simulink model "Candidacy_Exam_RR"  (R2023a)
settings: Solver=VariableStepAuto  StartTime=0  StopTime=1000  FixedStep=0.01  RelTol=1e-3
model workspace (MAT data in the model file):
  finalint = 0
  firstWarning = 1
  originalScenarioChecksum = '114339432DE22364D47BB28FC96DC10C'
undefined symbols (not defined in the file): Acceleration, ActorID, AngularVelocity, curvature, DefaultGear, Defined, DEND_B, DEND_S, DEND_T, direction, DiscIntNeverNeededParam, driving, Ego, EgoRefPose, gradbp, L, Lane, LF, LR, m, matlabshared, MAX_BRAKE, MAX_STEER, MAX_TORQUE, maxNumActors, MCAR, MIN_BRAKE, MIN_STEER, MIN_TORQUE, n, NUMD_B, NUMD_S, NUMD_T, Pitch, Pose, Position, psi_o, R, Roll, RRdamp, SceneInfo, session, sigbuilder_block, STEER_RATIO, stopSign_ID, Tdead, thetaRefs, TL_ID, TrackWidth, Ts, ts, User, Vdead, Velocity, WB, X_o, xRef2s, Y_o, Yaw, yRef2s
libraries: drivingscenarioandsensors x13, roadrunnerscenario x11, simulink x8, simulink_extras x5, drivingvehiclecontroller x2, trackingutilitieslib x2, robotalgslib x1, mpcadaslib x1, slpidlib x1, drivinglib x1, autolibshared x1, vehdynlibviscommon x1
(part 1 of 5)
settings Model: Creator=akshran  LastModifiedBy=moham
settings DataIOCC: SignalLogging=off
settings OptimizationCC: ReuseModelBlockBuffer=off
settings DebuggingCC: UnconnectedInputMsg=warning  UnconnectedOutputMsg=warning  UnconnectedLineMsg=warning  UnderSpecifiedDimensionMsg=warning
settings ModelReferenceCC: EnableRefExpFcnMdlSchedulingChecks=on
settings RTWCC: DLArmComputeVersion=19.05

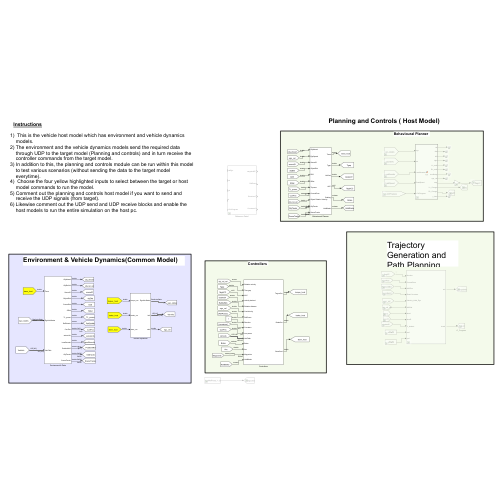
[thumbnail: Simulink's stored preview of the top-level diagram]
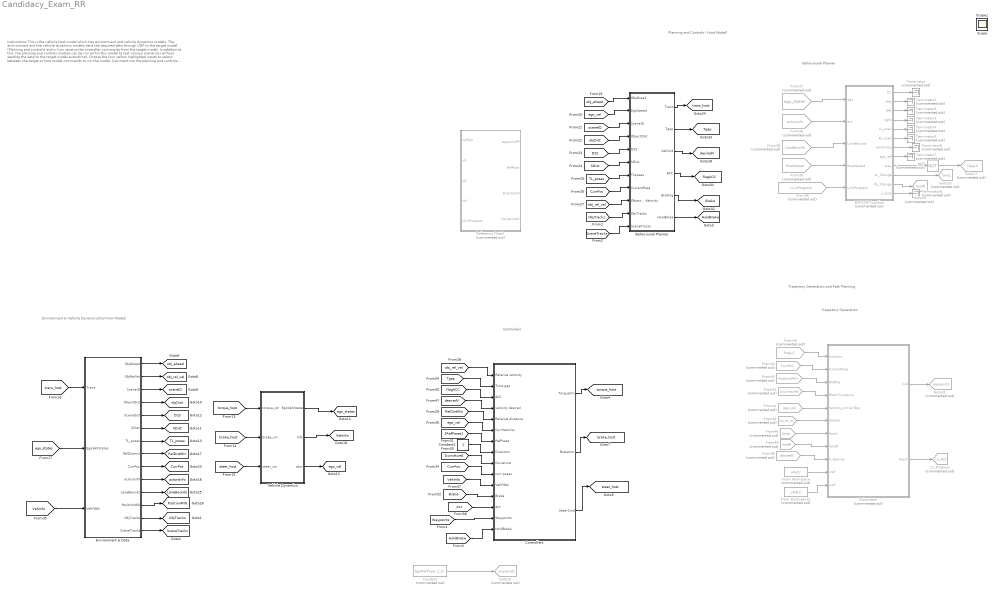
== system Candidacy_Exam_RR ==
  note: Trajectory Generation and Path Planning
  note: Trajectory Generation
  note: Behavioural Planner
  note: Instructions
      |
      | This is the vehicle host model which has environment and vehicle dynamics models.
      | The environment and the vehicle dynamics models send the required data through UDP to the target model (Planning and controls) and in turn receive the controller commands from the target model.
      | In addition to this, the planning and controls module can be run within this model to test various scenarios (without sending the data to the target model everytime).
      | Choose the four yellow highlighted inputs to select between the target or host model commands to run the model.
      | Comment out the planning and controls host model if you want to send and receive the UDP signals (from target).
      | Likewise comment out the UDP send and UDP receive blocks and enable the host models to run the entire simulation on the host pc.
  note: Environment & Vehicle Dynamics(Common Model)
  note: Planning and Controls ( Host Model)
  note: Controllers
  Behavioural Planner : Subsystem
  Constant : Constant  Commented=on  Value=EgoRefPose(:,1:2)
  Constant1 : Constant
  Controllers : Subsystem
  Environment & Data : Subsystem
  From Workspace : FromWorkspace  Commented=on  VariableName=xRef2
  From Workspace1 : FromWorkspace  Commented=on  VariableName=yRef2
  From36 : From  Commented=on  GotoTag=actorsInfo  TagVisibility=global
  From37 : From  Commented=on  GotoTag=ego_states  TagVisibility=global
  From38 : From  Commented=on  GotoTag=LaneBounds  TagVisibility=global
  From39 : From  Commented=on  GotoTag=RoadSpeed  TagVisibility=global
  From40 : From  Commented=on  GotoTag=CurrPos  TagVisibility=global
  From41 : From  Commented=on  GotoTag=curvature
  From42 : From  Commented=on  GotoTag=ego_vel  TagVisibility=global
  From43 : From  Commented=on  GotoTag=PositionMIO  TagVisibility=global
  From44 : From  Commented=on  GotoTag=obj_rel_vel  TagVisibility=global
  From45 : From  Commented=on  GotoTag=flagLC  TagVisibility=global
  From46 : From  Commented=on  GotoTag=laneL  TagVisibility=global
  From48 : From  Commented=on  GotoTag=desiredV  TagVisibility=global
  From49 : From  Commented=on  GotoTag=laneR  TagVisibility=global
  From56 : From  Commented=on  GotoTag=LCinProgress  TagVisibility=global
  Goto19 : Goto  Commented=on  GotoTag=waypoints  TagVisibility=global
  Goto21 : Goto  Commented=on  GotoTag=waypoints  TagVisibility=global
  Goto27 : Goto  Commented=on  GotoTag=flagLC  TagVisibility=global
  Goto29 : Goto  Commented=on  GotoTag=laneL  TagVisibility=global
  Goto30 : Goto  Commented=on  GotoTag=laneR  TagVisibility=global
  LC_Progress : Goto  Commented=on  GotoTag=LC_ACC  TagVisibility=global
  MATLAB Function : MATLAB Function  Commented=on  TreatAsAtomicUnit=on
  NOT : Logic  Commented=on  Operator=NOT  IconShape=distinctive  AllPortsSameDT=off  OutDataTypeStr=boolean
  Reference Data1 : Subsystem  Commented=on  VariantControl=Stanley
  Subsystem : Subsystem  Commented=on
  Terminator{,1..8} (9 alike) : Terminator  Commented=on
  Vehicle Dynamics : Subsystem
  Scope : Scope
  Scope1 : Scope
  tag scope: Brake=global, CurrPos=global, D2S=global, HoldBrake=global, LaneBounds=global, ObjTracks=global, PositionMIO=global, RelDistMin=global, SDist=global, SceneTracks=global, TL_poses=global, Tgap=global, VehInfo=global, actorsInfo=global, brake_host=global, desiredV=global, ego_states=global, ego_vel=global, flagACC=global, objDist=global, obj_ahead=global, obj_rel_vel=global, sceneID=global, steer_host=global, torque_host=global, trans_host=global
  wires:
  Controllers/1(TorgueCm) -> [torque_host]
  Environment & Data/1(ObjAhead) -> [obj_ahead]
  Environment & Data/2(ObjRelVel) -> [obj_rel_vel]
  Environment & Data/3(SceneID) -> [sceneID]
  Environment & Data/4(ObjectDist) -> [objDist]
  Environment & Data/6(SDist) -> [SDist]
  Environment & Data/5(SceneDist) -> [D2S]
  Environment & Data/7(TL_poses) -> [TL_poses]
  Vehicle Dynamics/1(EgoVehStates) -> [ego_states]
  Vehicle Dynamics/3(xdot) -> [ego_vel]
  Environment & Data/8(RelDistmin) -> [RelDistMin]
  Vehicle Dynamics/2(Info) -> [VehInfo]
  [torque_host] -> Vehicle Dynamics/1(torque_cm)
  [brake_host] -> Vehicle Dynamics/2(brake_cm)
  [steer_host] -> Vehicle Dynamics/3(steer_cm)
  [trans_host] -> Environment & Data/1(Trans)
  [ego_states] -> Environment & Data/2(EgoVehStates)
  [obj_rel_vel] -> Controllers/1(Relative velocity)
  [RelDistMin] -> Controllers/5(Relative distance)
  [ego_vel] -> Controllers/6(CurrVelocity)
  [RefPoses] -> Controllers/7(RefPoses)
  Constant1/1 -> Controllers/8(Direction)
  [curvature] -> Controllers/9(Curvature)
  [CurrPos] -> Controllers/10(curr poses)
  [VehInfo] -> Environment & Data/3(VehFdbk)
  Environment & Data/9(CurrPos) -> [CurrPos]
  Environment & Data/10(actorsinfo) -> [actorsInfo]
  From37/1 -> MATLAB Function/1(ego)
  From36/1 -> MATLAB Function/2(act)
  Environment & Data/11(LaneBounds) -> [LaneBounds]
  From38/1 -> MATLAB Function/3(LaneBounds)
  From39/1 -> MATLAB Function/4(RoadSpeed)
  MATLAB Function/9(stay) -> NOT/1
  MATLAB Function/10(LL_Change) -> Goto29/1
  MATLAB Function/11(RL_Change) -> Goto30/1
  Environment & Data/12(PositionMIO) -> [PositionMIO]
  NOT/1 -> Goto27/1
  [desiredV] -> Controllers/4(velocity desired)
  [Tgap] -> Controllers/2(Time gap)
  [flagACC] -> Controllers/3(ACC)
  From56/1 -> MATLAB Function/5(LCinProgress)
  [VehInfo] -> Controllers/11(VehFdbk)
  Controllers/2(BrakeCm) -> [brake_host]
  Controllers/3(SteerCmd) -> [steer_host]
  From45/1 -> Subsystem/1(function)
  From40/1 -> Subsystem/2(CurrentPose)
  From43/1 -> Subsystem/3(MIOPos)
  From41/1 -> Subsystem/4(Road Curvature)
  From42/1 -> Subsystem/5(Velocity_Initial_Ego)
  From44/1 -> Subsystem/6(MIOVel)
  From48/1 -> Subsystem/9(V_desired)
  Subsystem/2(check) -> LC_Progress/1
  [obj_ahead] -> Behavioural Planner/1(ObjAhead)
  [ego_vel] -> Behavioural Planner/2(EgoSpeed)
  [sceneID] -> Behavioural Planner/3(SceneID)
  [objDist] -> Behavioural Planner/4(ObjectDist)
  [D2S] -> Behavioural Planner/5(D2S)
  [SDist] -> Behavioural Planner/6(SDist)
  [TL_poses] -> Behavioural Planner/7(TLposes)
  [CurrPos] -> Behavioural Planner/8(CurrentPose)
  [obj_rel_vel] -> Behavioural Planner/9(Object Relative Velocity)
  Behavioural Planner/1(Trans) -> [trans_host]
  Behavioural Planner/2(Tgap) -> [Tgap]
  Behavioural Planner/3(VelCmd) -> [desiredV]
  Behavioural Planner/4(ACC) -> [flagACC]
  Behavioural Planner/5(Braking) -> [Brake]
  [Brake] -> Controllers/12(Brake)
  [Acc] -> Controllers/13(Acc)
  Subsystem/1(out) -> Goto21/1
  From46/1 -> Subsystem/7(laneL)
  From49/1 -> Subsystem/8(laneR)
  From Workspace/1 -> Subsystem/10(xref)
  From Workspace1/1 -> Subsystem/11(yref)
  MATLAB Function/1(ttc) -> Terminator/1
  MATLAB Function/2(dist) -> Terminator1/1
  MATLAB Function/3(left) -> Terminator2/1
  MATLAB Function/4(right) -> Terminator3/1
  MATLAB Function/5(LL_avail) -> Terminator4/1
  MATLAB Function/6(RL_avail) -> Terminator5/1
  MATLAB Function/7(tend2stay) -> Terminator6/1
  MATLAB Function/8(ego_vel) -> Terminator7/1
  MATLAB Function/12(y_lane) -> Terminator8/1
  Environment & Data/14(SceneTracks) -> [SceneTracks]
  Environment & Data/13(ObjTracks) -> [ObjTracks]
  [ObjTracks] -> Behavioural Planner/10(ObjTracks)
  [SceneTracks] -> Behavioural Planner/11(SceneTracks)
  Behavioural Planner/6(HoldBrake) -> [HoldBrake]
  [HoldBrake] -> Controllers/15(HoldBrake)
  Constant/1 -> Goto19/1
  [Waypoints] -> Controllers/14(Waypoints)

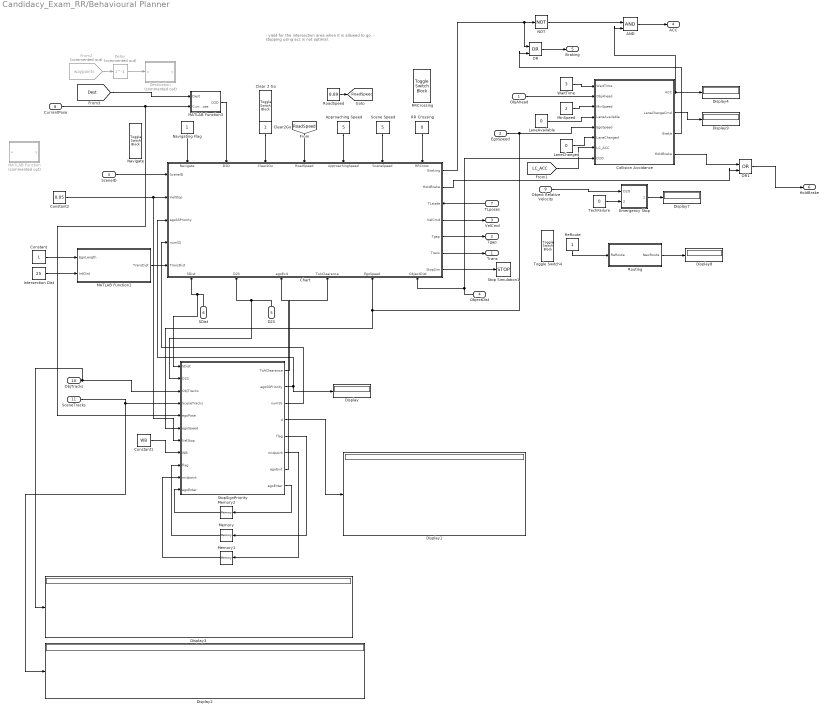
== system Candidacy_Exam_RR/Behavioural Planner ==
  note: - yield for the intersection area when it is allowed to go.
      | - stopping using acc is not optimal.
  ObjAhead : Inport
  EgoSpeed : Inport  Port=2
  SceneID : Inport  Port=3
  ObjectDist : Inport  Port=4
  D2S : Inport  Port=5
  SDist : Inport  Port=6
  TLposes : Inport  Port=7
  CurrentPose : Inport  Port=8
  Object Relative Velocity : Inport  Port=9
  ObjTracks : Inport  Port=10
  SceneTracks : Inport  Port=11
  AND : Logic  IconShape=distinctive  AllPortsSameDT=off  OutDataTypeStr=fixdt(1,16)
  Approaching Speed : Constant  Value=5
  Chart : Stateflow chart  TreatAsAtomicUnit=on
      settings: PortSchema="{\"entries\":[{\"content\":{\"sides\":[{\"content\":{\"connectorIds\":[\"In17\",\"In18\",\"In19\",\"In2\",\"In5\"]},\"type\":\"ConnectorPlacement.EquallySpacedRectSide\",\"uuid\":\"81aca70f-0947-49fb-b60a-be241e44193b\"},{\"content\":{\"connectorIds\":[\"Out6\",\"Out2\",\"In1\",\"Out1\",\"Out3\",\"Out4\",\"Out5\"],\"side\":\"RIGHT\"},\"type\":\"ConnectorPlacement.EquallySpacedRectSide\",\"uuid\":\"e7b9645e-3711-4964-ac9b-0199dd335e99\"},{\"content\":{\"connectorIds\":[\"In13\",\"In14\",\"In15\",\"In16\",\"In6\",\"In9\",\"In11\"],\"side\":\"TOP\"},\"type\":\"ConnectorPlacement.EquallySpacedRectSide\",\"uuid\":\"6876f024-944b-4540-9404-d68f37763657\"},{\"content\":{\"connectorIds\":[\"In10\",\"In12\",\"In3\",\"In4\",\"In7\",\"In8\"],\"side\":\"BOTTOM\"},\"type\":\"ConnectorPlacement.EquallySpacedRectSide\",\"uuid\":\"44acab73-cdde-4edf-95df-27422644ccab\"}]},\"type\":\"ConnectorPlacement.EquallySpacedConnector\",\"uuid\":\"d2c31c01-e447-43db-8d2b-8b98a0ca291a\"}],\"packageUris\":[\"http://schema.mathworks.com/mf0/Connector/R2020b\"],\"version\":\"1.0\"}"
  Clear 2 Go : ToggleSwitchBlock
      settings: Values={{'Off', 'On'}, [0 1]}
  Clear2Go : Constant
  Collision Avoidance : Stateflow chart  TreatAsAtomicUnit=on
  Constant : Constant  Value=L
  Constant1 : Constant  Value=WB
  Constant2 : Constant  Value=0.05
  Delay : Delay  Commented=on  DelayLength=1
  Destination : MATLAB Function  Commented=on  TreatAsAtomicUnit=on
  Display{,1..4,7..9} (8 alike) : Display
  Emergency Stop : Stateflow chart  TreatAsAtomicUnit=on
  From2 : From  Commented=on  GotoTag=waypoints  TagVisibility=global
  Intersection Dist : Constant  Value=25
  LaneAvailable : Constant  Value=0
  LaneChanged : Constant  Value=0
  MATLAB Function : MATLAB Function  Commented=on  TreatAsAtomicUnit=on
  MATLAB Function1 : MATLAB Function  TreatAsAtomicUnit=on
  MATLAB Function3 : MATLAB Function  TreatAsAtomicUnit=on
  Memory : Memory
  Memory1 : Memory  InitialCondition=[0 0]
  Memory2 : Memory
  MinSpeed : Constant  Value=2
  NOT : Logic  Operator=NOT  IconShape=distinctive  AllPortsSameDT=off  OutDataTypeStr=boolean
  Navigate : ToggleSwitchBlock
      settings: Values={{'Off', 'On'}, [0 1]}
  Navigating Flag : Constant
  OR : Logic  Operator=OR  IconShape=distinctive  AllPortsSameDT=off  OutDataTypeStr=boolean
  OR1 : Logic  Operator=OR  IconShape=distinctive  AllPortsSameDT=off  OutDataTypeStr=boolean
  RR Crossing : Constant  Value=0
  RRCrossing : ToggleSwitchBlock
      settings: Values={{'Off', 'On'}, [0 1]}
  ReRoute : Constant
  RoadSpeed : Constant  Value=8.89
  Routing : Stateflow chart  TreatAsAtomicUnit=on
  Scene Speed : Constant  Value=5
  Stop Simulation1 : Stop
  StopSignPriority : MATLAB Function  TreatAsAtomicUnit=on
  TechFailure : Constant  Value=0
  Toggle Switch4 : ToggleSwitchBlock
      settings: Values={{'Off', 'On'}, [0 1]}
  WaitTime : Constant  Value=3
  Trans : Outport
  Tgap : Outport  Port=2
  VelCmd : Outport  Port=3
  ACC : Outport  Port=4
  Braking : Outport  Port=5
  HoldBrake : Outport  Port=6
  tag scope: RoadSpeed=global
  wires:
  Clear2Go/1 -> Chart/15(Clear2Go)
  Routing/1(NewRoute) -> Display8/1
  ObjectDist/1 -> Chart/8(ObjectDist), Collision Avoidance/8(D2O)
  WaitTime/1 -> Collision Avoidance/1(WaitTime)
  Navigating Flag/1 -> Chart/13(Navigate)
  Approaching Speed/1 -> Chart/6(ApproachingSpeed)
  Scene Speed/1 -> Chart/9(SceneSpeed)
  EgoSpeed/1 -> Collision Avoidance/5(EgoSpeed), StopSignPriority/6(egoSpeed), Chart/7(EgoSpeed)
  ReRoute/1 -> Routing/1(ReRoute)
  Collision Avoidance/2(LaneChangeCmd) -> Display9/1
  LaneAvailable/1 -> Collision Avoidance/4(LaneAvailable)
  CurrentPose/1 -> StopSignPriority/5(egoPose), MATLAB Function3/2(CurrentPose)
  RR Crossing/1 -> Chart/11(RRCross)
  MinSpeed/1 -> Collision Avoidance/3(MinSpeed)
  LaneChanged/1 -> Collision Avoidance/6(LaneChanged)
  [RoadSpeed] -> Chart/16(RoadSpeed)
  ObjAhead/1 -> Collision Avoidance/2(ObjAhead)
  SceneID/1 -> Chart/17(SceneID)
  Chart/5(StopSim) -> Stop Simulation1/1
  Chart/4(Trans) -> Trans/1
  TLposes/1 -> Chart/1(TLstate)
  Chart/1(VelCmd) -> VelCmd/1
  SDist/1 -> Chart/10(SDist), StopSignPriority/1(SDist)
  D2S/1 -> Chart/12(D2S), StopSignPriority/2(D2S)
  Chart/3(Tgap) -> Tgap/1
  TechFailure/1 -> Emergency Stop/2(TechFailure)
  Emergency Stop/1(EStop) -> Display7/1
  Object Relative Velocity/1 -> Emergency Stop/1(D2O)
  Collision Avoidance/1(ACC) -> AND/2, Display4/1
  RoadSpeed/1 -> [RoadSpeed]
  NOT/1 -> AND/1
  AND/1 -> ACC/1
  Chart/6(Braking) -> OR/1, NOT/1
  OR/1 -> Braking/1
  Collision Avoidance/3(Brake) -> OR/2
  Constant/1 -> MATLAB Function1/1(EgoLength)
  Intersection Dist/1 -> MATLAB Function1/2(IntDist)
  MATLAB Function1/1(TransDist) -> Chart/5(TransDist)
  [LC_ACC] -> Collision Avoidance/7(LC_ACC)
  From2/1 -> Delay/1
  Delay/1 -> Destination/1(u)
  MATLAB Function3/1(D2D) -> Chart/14(D2D)
  Constant2/1 -> StopSignPriority/7(VelStop), Chart/18(VelStop)
  StopSignPriority/2(egoSSPriority) -> Display/1, Chart/19(egoSSPriority)
  SceneTracks/1 -> Display2/1, StopSignPriority/4(SceneTracks)
  ObjTracks/1 -> Display3/1, StopSignPriority/3(ObjTracks)
  StopSignPriority/3(numSS) -> Chart/2(numSS)
  Constant1/1 -> StopSignPriority/8(WB)
  StopSignPriority/4(d) -> Display1/1
  Memory/1 -> StopSignPriority/9("flag ")
  StopSignPriority/5(flag) -> Memory/1
  StopSignPriority/6(midpoint) -> Memory1/1
  Memory1/1 -> StopSignPriority/10("midpoint ")
  StopSignPriority/7(egoExit) -> Chart/3(egoExit)
  StopSignPriority/1(ToAClearance) -> Chart/4(ToAClearance)
  Chart/2(HoldBrake) -> OR1/2
  StopSignPriority/8(egoEnter) -> Memory2/1
  Memory2/1 -> StopSignPriority/11("egoEnter ")
  OR1/1 -> HoldBrake/1
  Collision Avoidance/4(HoldBrake) -> OR1/1
  [Dest] -> MATLAB Function3/1(Dest)

== system Candidacy_Exam_RR/Controllers ==
  note: Need to write code to get curvature Information
  Relative velocity : Inport
  Time gap : Inport  Port=2
  ACC : Inport  Port=3
  velocity desired : Inport  Port=4
  Relative distance : Inport  Port=5
  CurrVelocity : Inport  Port=6
  RefPoses : Inport  Port=7
  Direction : Inport  Port=8
  Curvature : Inport  Port=9
  curr poses : Inport  Port=10
  VehFdbk : Inport  Port=11
  Brake : Inport  Port=12
  Acc : Inport  Port=13
  Waypoints : Inport  Port=14
  HoldBrake : Inport  Port=15
  Lateral Controllers1 : Subsystem
  Longitudinal Controllers : Subsystem
  MATLAB Function2 : MATLAB Function  Commented=on  TreatAsAtomicUnit=on
  Subsystem1 : Subsystem
  Subsystem2 : Subsystem
      settings: PortSchema="{\"entries\":[{\"content\":{\"sides\":[{\"content\":{\"connectorIds\":[\"In1\",\"In2\",\"In3\",\"In4\"]},\"type\":\"ConnectorPlacement.EquallySpacedRectSide\",\"uuid\":\"a23b1a10-3bcb-40a0-900c-c9a3f160b173\"},{\"content\":{\"connectorIds\":[\"Out1\",\"Out2\"],\"side\":\"RIGHT\"},\"type\":\"ConnectorPlacement.EquallySpacedRectSide\",\"uuid\":\"88840b66-912f-4184-aeec-297642319416\"},{\"content\":{\"connectorIds\":[\"In5\",\"In6\",\"In7\",\"In8\"],\"side\":\"TOP\"},\"type\":\"ConnectorPlacement.EquallySpacedRectSide\",\"uuid\":\"37a03ca9-b065-473e-b290-3b07703c6005\"},{\"content\":{\"connectorIds\":[\"In9\",\"In10\"],\"side\":\"BOTTOM\"},\"type\":\"ConnectorPlacement.EquallySpacedRectSide\",\"uuid\":\"275ca825-7815-497a-af18-67b3ec4705b4\"}]},\"type\":\"ConnectorPlacement.EquallySpacedConnector\",\"uuid\":\"5bfc7c71-8f7a-4cba-a168-7eeca22a2fcb\"}],\"packageUris\":[\"http://schema.mathworks.com/mf0/Connector/R2020b\"],\"version\":\"1.0\"}"
  TorgueCm : Outport
  BrakeCm : Outport  Port=2
  SteerCmd : Outport  Port=3
  wires:
  Curvature/1 -> Lateral Controllers1/5(Curvature)
  Relative velocity/1 -> Longitudinal Controllers/2(Relative velocity)
  Direction/1 -> Longitudinal Controllers/7(Direction), Lateral Controllers1/4(Direction)
  RefPoses/1 -> Lateral Controllers1/3(RefPoses)
  CurrVelocity/1 -> Subsystem2/6(CurrVelocity), Longitudinal Controllers/1(Curr Velocity), Longitudinal Controllers/6(CurrVel), Lateral Controllers1/1(CurrVelocity)
  Time gap/1 -> Longitudinal Controllers/4(Time gap)
  Relative distance/1 -> Subsystem2/7(Relative Distance), Longitudinal Controllers/3(Relative distance)
  Subsystem1/2(PPpose) -> Lateral Controllers1/7(Pose)
  VehFdbk/1 -> Subsystem1/1(VehFdbk)
  Lateral Controllers1/1(steerCmd) -> SteerCmd/1
  velocity desired/1 -> Subsystem2/4(Set Velocity), Longitudinal Controllers/9(desiredVelocity), Longitudinal Controllers/5(Set velocity)
  curr poses/1 -> Lateral Controllers1/2(CurrPoses), Longitudinal Controllers/10(CurrentPose)
  Longitudinal Controllers/1(Longitudinal acceleration) -> Subsystem2/1(ACCaccel_cmd)
  Longitudinal Controllers/2(AccelCmd) -> Subsystem2/2(LCaccel_cmd)
  Longitudinal Controllers/3(DecelCmd) -> Subsystem2/3(LCdeccel_cmd)
  ACC/1 -> Subsystem2/5(ACC)
  Subsystem2/1(TorgueCm) -> TorgueCm/1
  Subsystem2/2(BrakeCm) -> BrakeCm/1
  Acc/1 -> Subsystem2/9(CurrAccel), Longitudinal Controllers/11(Current Accel)
  Brake/1 -> Subsystem2/8(Braking), Longitudinal Controllers/12(Brake)
  Waypoints/1 -> Longitudinal Controllers/8(RefXY), Lateral Controllers1/6(Waypoints)
  HoldBrake/1 -> Subsystem2/10(HoldBrake)

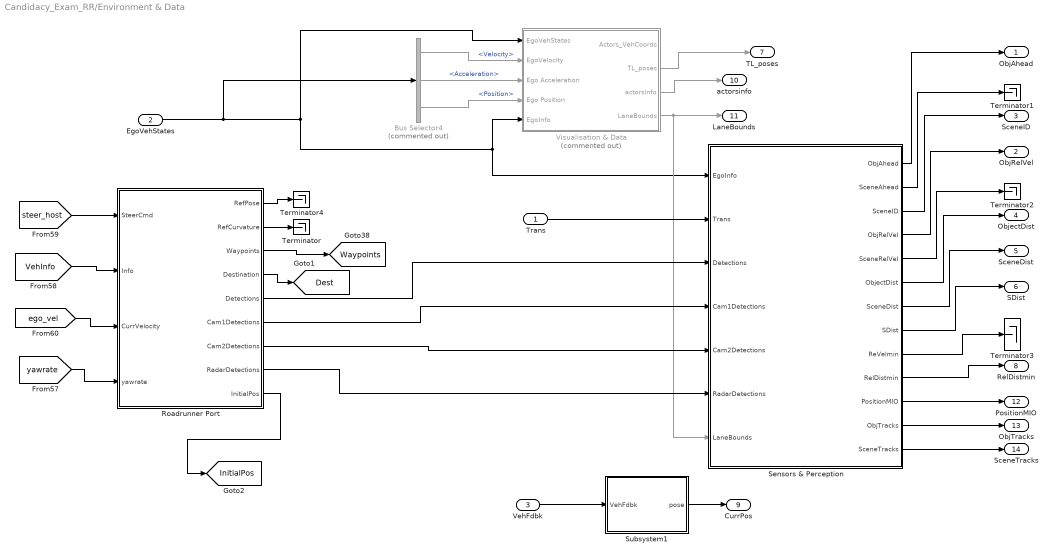
== system Candidacy_Exam_RR/Environment & Data ==
  Trans : Inport
  EgoVehStates : Inport  Port=2
  VehFdbk : Inport  Port=3
  Bus Selector4 : BusSelector  Commented=on  OutputSignals=Velocity,Acceleration,Position
  Roadrunner Port : Subsystem
  Sensors & Perception : Subsystem
  Subsystem1 : Subsystem
  Terminator{,1..4} (5 alike) : Terminator
  Visualisation & Data : Subsystem  Commented=on
  ObjAhead : Outport
  ObjRelVel : Outport  Port=2
  SceneID : Outport  Port=3
  ObjectDist : Outport  Port=4
  SceneDist : Outport  Port=5
  SDist : Outport  Port=6
  TL_poses : Outport  Port=7
  RelDistmin : Outport  Port=8
  CurrPos : Outport  Port=9
  actorsinfo : Outport  Port=10
  LaneBounds : Outport  Port=11
  PositionMIO : Outport  Port=12
  ObjTracks : Outport  Port=13
  SceneTracks : Outport  Port=14
  tag scope: Dest=global, InitialPos=global, Waypoints=global
  wires:
  Sensors & Perception/11(PositionMIO) -> PositionMIO/1
  Sensors & Perception/3(SceneID) -> SceneID/1
  Subsystem1/1(pose) -> CurrPos/1
  Sensors & Perception/5(SceneRelVel) -> Terminator2/1
  EgoVehStates/1 -> Sensors & Perception/1(EgoInfo), Visualisation & Data/5(EgoInfo), Visualisation & Data/1(EgoVehStates), Bus Selector4/1
  VehFdbk/1 -> Subsystem1/1(VehFdbk)
  Bus Selector4/2 -> Visualisation & Data/3(Ego Acceleration)  "<Acceleration>"
  Bus Selector4/1 -> Visualisation & Data/2(EgoVelocity)  "<Velocity>"
  Visualisation & Data/2(TL_poses) -> TL_poses/1
  Bus Selector4/3 -> Visualisation & Data/4(Ego Position)  "<Position>"
  Visualisation & Data/3(actorsinfo) -> actorsinfo/1
  Visualisation & Data/4(LaneBounds) -> Sensors & Perception/7(LaneBounds), LaneBounds/1
  Trans/1 -> Sensors & Perception/2(Trans)
  Sensors & Perception/9(ReVelmin) -> Terminator3/1
  Sensors & Perception/1(ObjAhead) -> ObjAhead/1
  Sensors & Perception/10(RelDistmin) -> RelDistmin/1
  Sensors & Perception/2(SceneAhead) -> Terminator1/1
  Sensors & Perception/4(ObjRelVel) -> ObjRelVel/1
  Sensors & Perception/6(ObjectDist) -> ObjectDist/1
  Sensors & Perception/7(SceneDist) -> SceneDist/1
  Sensors & Perception/8(SDist) -> SDist/1
  Sensors & Perception/12(ObjTracks) -> ObjTracks/1
  Sensors & Perception/13(SceneTracks) -> SceneTracks/1
  Roadrunner Port/8(RadarDetections) -> Sensors & Perception/6(RadarDetections)
  [VehInfo] -> Roadrunner Port/2(Info)
  Roadrunner Port/9(InitialPos) -> [InitialPos]
  Roadrunner Port/7(Cam2Detections) -> Sensors & Perception/5(Cam2Detections)
  [ego_vel] -> Roadrunner Port/3(CurrVelocity)
  [yawrate] -> Roadrunner Port/4(yawrate)
  Roadrunner Port/1(RefPose) -> Terminator4/1
  Roadrunner Port/2(RefCurvature) -> Terminator/1
  Roadrunner Port/3(Waypoints) -> [Waypoints]
  Roadrunner Port/6(Cam1Detections) -> Sensors & Perception/4(Cam1Detections)
  [steer_host] -> Roadrunner Port/1(SteerCmd)
  Roadrunner Port/5(Detections) -> Sensors & Perception/3(Detections)
  Roadrunner Port/4(Destination) -> [Dest]

== system Candidacy_Exam_RR/Reference Data1 ==
  velEgo : Inport
  xd : Inport  Port=2
  yd : Inport  Port=3
  In4 : Inport  Port=4
  LCinProgress : Inport  Port=5
  Discrete-Time Integrator : DiscreteIntegrator  SampleTime=-1  ICPrevOutput=DiscIntNeverNeededParam  ICPrevScaledInput=DiscIntNeverNeededParam
  Memory : Memory
  Memory1 : Memory
  Merge : Merge
  Merge1 : Merge
  Subsystem : Subsystem
  Subsystem1 : Subsystem
  Subsystem2 : Subsystem
  Subsystem3 : Subsystem
  Switch : Switch  Criteria=u2 ~= 0  SaturateOnIntegerOverflow=off  InputSameDT=off
  Switch Case : SwitchCase  CaseConditions={1,0}  ShowDefaultCase=off
  waypointPP : Outport
  RefPose : Outport  Port=2
  DirectionO : Outport  Port=3
  CurvatureO : Outport  Port=4
  wires:
  velEgo/1 -> Subsystem3/1(VelFdbk), Subsystem2/1(VelFdbk), Discrete-Time Integrator/1
  Subsystem2/4(WayPoints) -> Merge1/1
  Merge1/1 -> waypointPP/1
  Subsystem2/1(RefPose) -> Switch/3
  Subsystem2/2(DirectionO) -> DirectionO/1
  Merge/1 -> CurvatureO/1
  Subsystem2/3(CurvatureO) -> Merge/2
  Subsystem3/1(RefPose) -> Switch/1
  Switch Case/1 -> Subsystem3/Action
  Switch Case/2 -> Subsystem2/Action
  xd/1 -> Memory/1
  yd/1 -> Memory1/1
  Memory/1 -> Subsystem3/2(xd)
  Memory1/1 -> Subsystem3/4(yd)
  Subsystem2/5(finalint) -> Subsystem3/3(finalint)
  Subsystem/1(Out1) -> Switch/2, Switch Case/1, Subsystem1/2(enable)
  LCinProgress/1 -> Subsystem/Enable
  Discrete-Time Integrator/1 -> Subsystem1/1(Integrator)
  Subsystem1/1(Ref pose) -> RefPose/1

== system Candidacy_Exam_RR/Subsystem ==
  function : Inport
  CurrentPose : Inport  Port=2
  MIOPos : Inport  Port=3
  Road Curvature : Inport  Port=4
  Velocity_Initial_Ego : Inport  Port=5
  MIOVel : Inport  Port=6
  laneL : Inport  Port=7
  laneR : Inport  Port=8
  V_desired : Inport  Port=9
  xref : Inport  Port=10
  yref : Inport  Port=11
  Delay : Delay  DelayLength=1
  Function-Call Subsystem : Subsystem  TreatAsAtomicUnit=on
  PathPlanner : Subsystem
  Terminator : Terminator
  To Workspace2 : ToWorkspace  VariableName=xd  SampleTime=-1
      settings: Save2DSignal=2-D array (concatenate along first dimension)
  To Workspace3 : ToWorkspace  VariableName=yd  SampleTime=-1
      settings: Save2DSignal=2-D array (concatenate along first dimension)
  Turns LC in prog off : MATLAB Function  TreatAsAtomicUnit=on
  out : Outport
  check : Outport  Port=2
  tag scope: LCinProgress=global, xd=global, yd=global
  wires:
  MIOVel/1 -> Function-Call Subsystem/5(MIOVel)
  Road Curvature/1 -> Function-Call Subsystem/3(Road Curvature)
  PathPlanner/1(out) -> out/1
  PathPlanner/2(check) -> check/1
  Velocity_Initial_Ego/1 -> Function-Call Subsystem/4(Velocity_Initial_Ego)
  V_desired/1 -> Function-Call Subsystem/6(V_desired)
  MIOPos/1 -> Function-Call Subsystem/2(MIOPos)
  Function-Call Subsystem/1(xd) -> To Workspace2/1, PathPlanner/2(xd), [xd]
  Function-Call Subsystem/2(yd) -> PathPlanner/5(yd), [yd], To Workspace3/1
  Delay/1 -> Turns LC in prog off/1(u)
  Turns LC in prog off/1(y) -> [LCinProgress]
  Function-Call Subsystem/3(LCinProgress) -> Delay/1
  CurrentPose/1 -> PathPlanner/1(CurrentPose), Function-Call Subsystem/1(EgoPosition)
  function/1 -> Function-Call Subsystem/Trigger
  laneL/1 -> Function-Call Subsystem/7(laneL)
  laneR/1 -> Function-Call Subsystem/8(laneR)
  xref/1 -> PathPlanner/3(xref)
  yref/1 -> PathPlanner/4(yref)
  PathPlanner/3(dcheck) -> Terminator/1
  [flagLC] -> PathPlanner/6(LC)

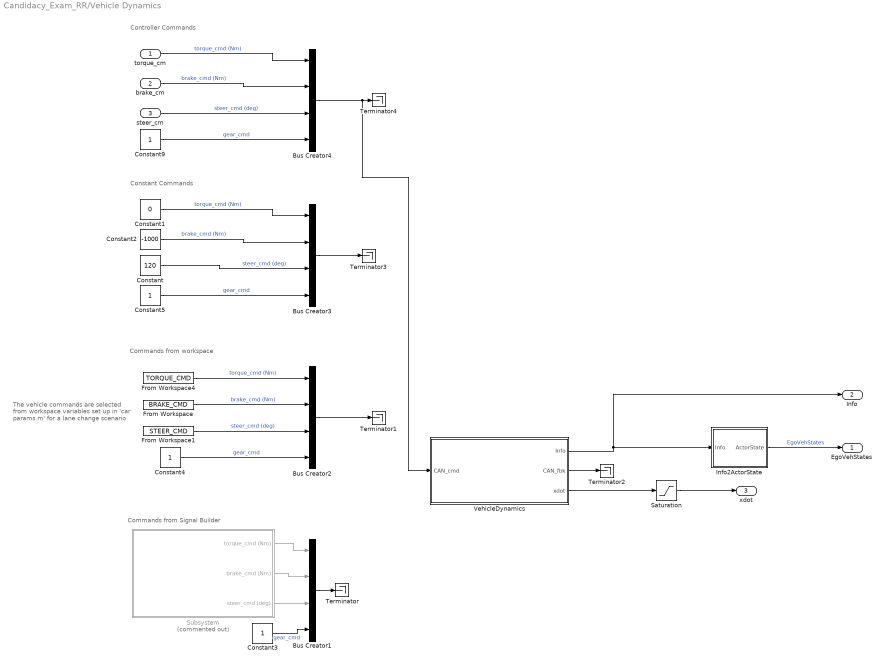
== system Candidacy_Exam_RR/Vehicle Dynamics ==
  note: Constant Commands
  note: Commands from workspace
  note: Commands from Signal Builder
  note: The vehicle commands are selected from workspace variables set up in 'car params.m' for a lane change scenario
  note: Controller Commands
  torque_cm : Inport
  brake_cm : Inport  Port=2
  steer_cm : Inport  Port=3
  Bus Creator{1..4} (4 alike) : BusCreator  Inputs=4
  Constant : Constant  Value=120
  Constant1 : Constant  Value=0
  Constant2 : Constant  Value=-1000
  Constant{3..5,9} (4 alike) : Constant
  From Workspace : FromWorkspace  VariableName=BRAKE_CMD  SampleTime=ts
  From Workspace1 : FromWorkspace  VariableName=STEER_CMD  SampleTime=ts
  From Workspace4 : FromWorkspace  VariableName=TORQUE_CMD  SampleTime=ts
  Info2ActorState : Subsystem
  Saturation : Saturate  UpperLimit=inf  LowerLimit=0.001
  Subsystem : Subsystem  Commented=on
  Terminator{,1..4} (5 alike) : Terminator
  VehicleDynamics : Subsystem  mask{InitPosition=[X_o Y_o 0]*0, InitSpeed=0, InitYaw=psi_o}
      mask prompts: InitPosition "Initial Position (m)"; InitSpeed "Initial Speed (m/s)"; InitYaw "Init Yaw (rad)"
  EgoVehStates : Outport
  Info : Outport  Port=2
  xdot : Outport  Port=3
  wires:
  Bus Creator2/1 -> Terminator1/1
  VehicleDynamics/2(CAN_fbk) -> Terminator2/1
  VehicleDynamics/1(Info) -> Info/1, Info2ActorState/1(Info)
  Constant/1 -> Bus Creator3/3  "steer_cmd (deg)"
  Info2ActorState/1(ActorState) -> EgoVehStates/1  "EgoVehStates"
  Constant1/1 -> Bus Creator3/1  "torque_cmd (Nm)"
  Constant2/1 -> Bus Creator3/2  "brake_cmd (Nm)"
  VehicleDynamics/3(xdot) -> Saturation/1
  Subsystem/1(torque_cmd (Nm)) -> Bus Creator1/1
  Subsystem/2(brake_cmd (Nm)) -> Bus Creator1/2
  Subsystem/3(steer_cmd (deg)) -> Bus Creator1/3
  Constant3/1 -> Bus Creator1/4  "gear_cmd"
  Constant4/1 -> Bus Creator2/4  "gear_cmd"
  From Workspace/1 -> Bus Creator2/2  "brake_cmd (Nm)"
  From Workspace1/1 -> Bus Creator2/3  "steer_cmd (deg)"
  From Workspace4/1 -> Bus Creator2/1  "torque_cmd (Nm)"
  Constant5/1 -> Bus Creator3/4  "gear_cmd"
  Bus Creator1/1 -> Terminator/1
  brake_cm/1 -> Bus Creator4/2  "brake_cmd (Nm)"
  Constant9/1 -> Bus Creator4/4  "gear_cmd"
  torque_cm/1 -> Bus Creator4/1  "torque_cmd (Nm)"
  steer_cm/1 -> Bus Creator4/3  "steer_cmd (deg)"
  Bus Creator3/1 -> Terminator3/1
  Bus Creator4/1 -> VehicleDynamics/1(CAN_cmd), Terminator4/1
  Saturation/1 -> xdot/1

== system Candidacy_Exam_RR/Controllers/Lateral Controllers1 ==
  note: include toggle logic
  CurrVelocity : Inport
  CurrPoses : Inport  Port=2
  RefPoses : Inport  Port=3
  Direction : Inport  Port=4
  Curvature : Inport  Port=5
  Waypoints : Inport  Port=6
  Pose : Inport  Port=7
  Constant : Constant  Commented=on
  Demux : Demux  Commented=on  Outputs=3
  Demux1 : Demux  Commented=on  Outputs=3
  From : From  Commented=on  GotoTag=yawrate  TagVisibility=global
  Gain : Gain  Gain=1/STEER_RATIO
  Gain1 : Gain  Commented=on  Gain=180/pi
  Gain2 : Gain  Gain=180/pi
  Lateral Controller Stanley : drivingvehiclecontroller/Lateral Controller Stanley  Commented=on  ModelType=Kinematic bicycle model  PositionGainF=0.75  PositionGainR=2.5  YawRateGain=0.05  DelayGain=0.05  VehicleMass=MCAR  Lf=LF  Lr=LR  TireStiffness=5e3  Wheelbase=3  MaxSteeringAngle=30
  Pure Pursuit Controller1 : Subsystem
  Scope2 : Scope  Commented=on  NumInputPorts=2
  Unit Delay : UnitDelay  Commented=on  SampleTime=-1  HasFrameUpgradeWarning=on
  steerCmd : Outport
  wires:
  From/1 -> Gain1/1
  CurrPoses/1 -> Demux1/1, Lateral Controller Stanley/2
  Pure Pursuit Controller1/1(delta) -> Gain2/1
  Gain/1 -> steerCmd/1
  Curvature/1 -> ?
  CurrVelocity/1 -> Lateral Controller Stanley/3
  RefPoses/1 -> Demux/1, Lateral Controller Stanley/1
  Pose/1 -> Pure Pursuit Controller1/1(Pose)
  Lateral Controller Stanley/1 -> Unit Delay/1
  Constant/1 -> Lateral Controller Stanley/4
  Demux1/2 -> Scope2/2
  Demux/2 -> Scope2/1
  Gain2/1 -> Gain/1
  Waypoints/1 -> Pure Pursuit Controller1/2(Waypoints)

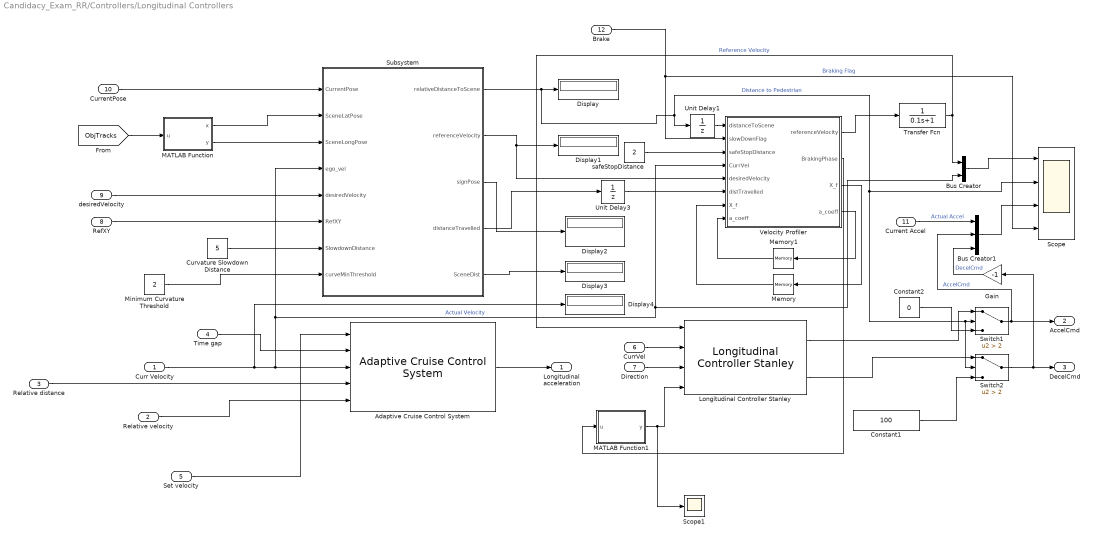
== system Candidacy_Exam_RR/Controllers/Longitudinal Controllers ==
  Curr Velocity : Inport
  Relative velocity : Inport  Port=2
  Relative distance : Inport  Port=3
  Time gap : Inport  Port=4
  Set velocity : Inport  Port=5
  CurrVel : Inport  Port=6
  Direction : Inport  Port=7
  RefXY : Inport  Port=8
  desiredVelocity : Inport  Port=9
  CurrentPose : Inport  Port=10
  Current Accel : Inport  Port=11
  Brake : Inport  Port=12
  Adaptive Cruise Control System : mpcadaslib/Adaptive Cruise Control System  EgoModel=tf(1,[0.5,1,0])  InitialEgoVelocity=0  DefaultSpacing=WB+2  MaxVelocity=50  MinAcceleration=-40  amin_ext=off  MaxAcceleration=40  amax_ext=off  Ts=0.1  PredictionHorizon=10  ControllerBehavior=1.0  suboptimal=off  maxiter=10  datatypeopt=double  optmode=off  trackmode=off
  Bus Creator : BusCreator  Inputs=2
  Bus Creator1 : BusCreator  Inputs=3
  Constant1 : Constant  Value=100
  Constant2 : Constant  Value=0
  Curvature Slowdown Distance : Constant  Value=5
  Display{,1..4} (5 alike) : Display
  Gain : Gain  Gain=-1
  Longitudinal Controller Stanley : drivingvehiclecontroller/Longitudinal Controller Stanley  Kp=1.9  Ki=1.4  SampleTime=0.05  MaxAcceleration=2  MaxDeceleration=2.1
  MATLAB Function : MATLAB Function  TreatAsAtomicUnit=on
  MATLAB Function1 : MATLAB Function  TreatAsAtomicUnit=on
  Memory : Memory  InheritSampleTime=on
  Memory1 : Memory  InitialCondition=zeros(6,1)  InheritSampleTime=on
  "Minimum Curvature Threshold " : Constant  Value=2
  Scope : Scope  NumInputPorts=4
  Scope1 : Scope
  Subsystem : Subsystem
  Switch1 : Switch  Criteria=u2 > Threshold  Threshold=2  SaturateOnIntegerOverflow=off  InputSameDT=off
  Switch2 : Switch  Criteria=u2 > Threshold  Threshold=2  SaturateOnIntegerOverflow=off  InputSameDT=off
  Transfer Fcn : TransferFcn  Denominator=[0.1 1]
  Unit Delay1 : UnitDelay  SampleTime=-1  HasFrameUpgradeWarning=on
  Unit Delay3 : UnitDelay  SampleTime=-1  HasFrameUpgradeWarning=on
  Velocity Profiler : MATLAB Function  TreatAsAtomicUnit=on
  safeStopDistance : Constant  Value=2
  Longitudinal acceleration : Outport
  AccelCmd : Outport  Port=2
  DecelCmd : Outport  Port=3
  wires:
  Set velocity/1 -> Adaptive Cruise Control System/1
  Curr Velocity/1 -> Display4/1, Subsystem/4(ego_vel), Bus Creator/2, Velocity Profiler/4(CurrVel), Adaptive Cruise Control System/3  "Actual Velocity"
  CurrVel/1 -> Longitudinal Controller Stanley/2
  Longitudinal Controller Stanley/2 -> Switch2/1
  Relative velocity/1 -> Adaptive Cruise Control System/5
  Relative distance/1 -> Adaptive Cruise Control System/4
  Adaptive Cruise Control System/1 -> Longitudinal acceleration/1
  Time gap/1 -> Adaptive Cruise Control System/2
  Direction/1 -> Longitudinal Controller Stanley/3
  Curvature Slowdown Distance/1 -> Subsystem/7(SlowdownDistance)
  "Minimum Curvature Threshold "/1 -> Subsystem/8(curveMinThreshold)
  RefXY/1 -> Subsystem/6(RefXY)
  desiredVelocity/1 -> Subsystem/5(desiredVelocity)
  CurrentPose/1 -> Subsystem/1(CurrentPose)
  [ObjTracks] -> MATLAB Function/1(u)
  MATLAB Function/1(x) -> Subsystem/2(SceneLatPose)
  MATLAB Function/2(y) -> Subsystem/3(SceneLongPose)
  Subsystem/1(relativeDistanceToScene) -> Unit Delay1/1, Switch2/2, Switch1/2, Scope/2, Display/1  "Distance to Pedestrian"
  Subsystem/3(signPose) -> Display2/1
  Brake/1 -> Velocity Profiler/2(slowDownFlag), Scope/4  "Braking Flag"
  safeStopDistance/1 -> Velocity Profiler/3(safeStopDistance)
  Velocity Profiler/1(referenceVelocity) -> Transfer Fcn/1
  Constant1/1 -> Switch2/3
  Switch2/1 -> Gain/1, DecelCmd/1
  Switch1/1 -> Bus Creator1/2, AccelCmd/1  "AccelCmd"
  Longitudinal Controller Stanley/1 -> Switch1/1
  Constant2/1 -> Switch1/3
  Bus Creator/1 -> Scope/1
  Subsystem/4(distanceTravelled) -> Unit Delay3/1
  Current Accel/1 -> Bus Creator1/1  "Actual Accel"
  Bus Creator1/1 -> Scope/3
  Gain/1 -> Bus Creator1/3  "DecelCmd"
  Transfer Fcn/1 -> Bus Creator/1, Longitudinal Controller Stanley/1  "Reference Velocity"
  Unit Delay3/1 -> Velocity Profiler/6(distTravelled)
  Subsystem/2(referenceVelocity) -> Velocity Profiler/5(desiredVelocity), Display1/1
  Velocity Profiler/4(a_coeff) -> Memory1/1
  Memory1/1 -> Velocity Profiler/8("a_coeff ")
  Velocity Profiler/3(X_f) -> Memory/1
  Memory/1 -> Velocity Profiler/7("X_f ")
  Unit Delay1/1 -> Velocity Profiler/1(distanceToScene)
  Subsystem/5(SceneDist) -> Display3/1
  Velocity Profiler/2(BrakingPhase) -> MATLAB Function1/1(u)
  MATLAB Function1/1(y) -> Scope1/1, Longitudinal Controller Stanley/4

== system Candidacy_Exam_RR/Controllers/Subsystem1 ==
  VehFdbk : Inport
  Bus Selector : BusSelector  OutputSignals=InertFrm.Cg.Disp.X,InertFrm.Cg.Disp.Y,InertFrm.Cg.Ang.psi
  Bus Selector1 : BusSelector  Commented=on  OutputSignals=InertFrm.Cg.Disp.X,InertFrm.Cg.Disp.Y,InertFrm.Cg.Disp.Z
  Gain1 : Gain  Gain=180/pi
  Mux : Mux  Inputs=3
  Mux1 : Mux  Commented=on  Inputs=3
  Mux2 : Mux  Inputs=3
  Transpose : Math  Operator=transpose  SignedPower=on
  Transpose1 : Math  Commented=on  Operator=transpose  SignedPower=on
  Transpose2 : Math  Operator=transpose  SignedPower=on
  pose : Outport
  PPpose : Outport  Port=2
  wires:
  Mux/1 -> Transpose/1
  VehFdbk/1 -> Bus Selector1/1, Bus Selector/1
  Gain1/1 -> Mux/3
  Transpose/1 -> pose/1
  Bus Selector/3 -> Mux2/3, Gain1/1  "<psi>"
  Bus Selector1/1 -> Mux1/1  "<X>"
  Bus Selector1/2 -> Mux1/2  "<Y>"
  Bus Selector1/3 -> Mux1/3  "<Z>"
  Mux1/1 -> Transpose1/1
  Mux2/1 -> Transpose2/1
  Transpose2/1 -> PPpose/1
  Bus Selector/2 -> Mux/2, Mux2/2  "<Y>"
  Bus Selector/1 -> Mux/1, Mux2/1  "<X>"

== system Candidacy_Exam_RR/Controllers/Subsystem2 ==
  ACCaccel_cmd : Inport
  LCaccel_cmd : Inport  Port=2
  LCdeccel_cmd : Inport  Port=3
  Set Velocity : Inport  Port=4
  ACC : Inport  Port=5
  CurrVelocity : Inport  Port=6
  Relative Distance : Inport  Port=7
  Braking : Inport  Port=8
  CurrAccel : Inport  Port=9
  HoldBrake : Inport  Port=10
  Constant : Constant  Value=0
  MATLAB Function : MATLAB Function  TreatAsAtomicUnit=on
  Subsystem : Subsystem
      settings: PortSchema="{\"entries\":[{\"content\":{\"sides\":[{\"content\":{\"connectorIds\":[\"In1\",\"In2\",\"In3\",\"In4\",\"In5\"]},\"type\":\"ConnectorPlacement.EquallySpacedRectSide\",\"uuid\":\"6c9a9437-5364-4180-a50b-e6d6b79cdde7\"},{\"content\":{\"connectorIds\":[\"Out1\"],\"side\":\"RIGHT\"},\"type\":\"ConnectorPlacement.EquallySpacedRectSide\",\"uuid\":\"0c9d90ab-7b55-4efa-a55f-4d6656a67f49\"},{\"content\":{\"side\":\"TOP\"},\"type\":\"ConnectorPlacement.EquallySpacedRectSide\",\"uuid\":\"ae5230ee-a902-425c-beff-008108cd3a63\"},{\"content\":{\"connectorIds\":[\"In6\"],\"side\":\"BOTTOM\"},\"type\":\"ConnectorPlacement.EquallySpacedRectSide\",\"uuid\":\"84107842-f68a-411d-a329-d9554f488760\"}]},\"type\":\"ConnectorPlacement.EquallySpacedConnector\",\"uuid\":\"1e045dad-e983-4ca4-b515-afd5db4fa0f5\"}],\"packageUris\":[\"http://schema.mathworks.com/mf0/Connector/R2020b\"],\"version\":\"1.0\"}"
  Subsystem1 : Subsystem
  Switch{,1..3} (4 alike) : Switch  Criteria=u2 > Threshold  SaturateOnIntegerOverflow=off  InputSameDT=off
  TorgueCm : Outport
  BrakeCm : Outport  Port=2
  wires:
  Subsystem1/2(brake_cm) -> BrakeCm/1, Switch2/3
  Subsystem1/1(torque_cm) -> TorgueCm/1, Switch3/3
  ACCaccel_cmd/1 -> MATLAB Function/1(u)
  ACC/1 -> Switch1/2, Switch/2
  MATLAB Function/1(accel) -> Switch/1
  LCaccel_cmd/1 -> Subsystem1/1(acc_cmd), Switch/3
  LCdeccel_cmd/1 -> Subsystem1/2(decc_cmd), Switch1/3
  MATLAB Function/2(decel) -> Switch1/1
  Constant/1 -> Switch3/1
  Braking/1 -> Switch3/2, Switch2/2, Subsystem/4("Braking ")
  CurrVelocity/1 -> Subsystem/1(CurrVelocity)
  Relative Distance/1 -> Subsystem/2(Relative Distance)
  Subsystem/1(BrakeCm) -> Switch2/1
  CurrAccel/1 -> Subsystem/3(CurrAccel)
  Set Velocity/1 -> Subsystem/5(Set Velocity)
  HoldBrake/1 -> Subsystem/6(HoldBrake)
